simulink model "Revolution_Current_Double_Loop_math"  (Simulink 7.5)
settings: Solver=ode15s  StartTime=0.0  StopTime=6  RelTol=1e-3
libraries: simulink x1, powerlib x1
settings Model: Creator=lm  LastModifiedBy=lm

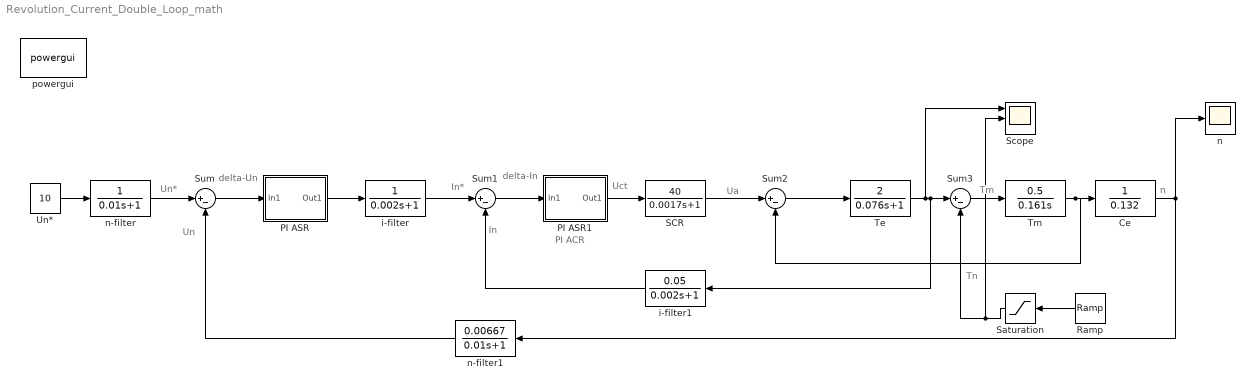
== system Revolution_Current_Double_Loop_math ==
  note: Tm
  note: n
  note: Tn
  note: Un*
  note: Un
  note: delta-Un
  note: In*
  note: In
  note: delta-In
  note: Uct
  note: Ua
  note: PI ACR
  Ce : TransferFcn  Denominator=[0 0.132]
  PI ASR : Subsystem
  PI ASR1 : Subsystem
  Ramp : simulink/Sources/Ramp  SystemSampleTime=-1  slope=1000  start=0.8  X0=0
  SCR : TransferFcn  Numerator=40  Denominator=[0.0017 1]
  Saturation : Saturate  UpperLimit=2222  OutDataType=fixdt(1, 16)  OutScaling=2^0
  Scope : Scope  NumInputPorts=3
      settings: YMin=-5~-5~-5  YMax=5~5~5
  Sum{,1..3} (4 alike) : Sum  Inputs=|+-  OutDataType=fixdt(1, 16)  OutScaling=2^0
  Te : TransferFcn  Numerator=[2]  Denominator=[0.076 1]
  Tm : TransferFcn  Numerator=[0.5]  Denominator=[0.161 0]
  Un* : Constant  Value=10  OutDataType=fixdt(1, 16)  OutScaling=2^0
  i-filter : TransferFcn  Denominator=[0.002 1]
  i-filter1 : TransferFcn  Numerator=0.05  Denominator=[0.002 1]
  n : Scope
  n-filter : TransferFcn  Denominator=[0.01 1]
  n-filter1 : TransferFcn  Numerator=[0.00667]  Denominator=[0.01 1]
  powergui : powerlib/powergui  Priority=1  SystemSampleTime=-1  SimulationMode=Discrete  SampleTime=50e-6  frequency=60  SPID=off  DisableSnubberDevices=off  DisableRonSwitches=off  DisableVfSwitches=off  SwTol=0  Interpol=off  frequencyindice=0  echomessages=off  HookPort=off  DisplayEquations=off  FunctionMessages=off  EnableUseOfTLC=off  x0status=blocks  RestoreLinks=warning  ResistiveCurrentMeasurement=off  Ylog=off  Xlog=on  ShowGrid=off  save=off  variable=ZData  ZoomFFT=off  StartTime=0.0  cycles=1  DisplayStyle=1  FreqAxis=off  MaxFrequency=1000  frequencyindicesteady=1  display=off  methode=off
  wires:
  Un*/1 -> n-filter/1
  n-filter/1 -> Sum/1
  Sum/1 -> PI ASR/1(In1)
  PI ASR/1(Out1) -> i-filter/1
  i-filter/1 -> Sum1/1
  Sum1/1 -> PI ASR1/1(In1)
  PI ASR1/1(Out1) -> SCR/1
  SCR/1 -> Sum2/1
  Te/1 -> Scope/1, Sum3/1, i-filter1/1
  Sum3/1 -> Tm/1
  Tm/1 -> Ce/1, Sum2/2
  Ce/1 -> n/1, n-filter1/1
  i-filter1/1 -> Sum1/2
  Saturation/1 -> Sum3/2, Scope/2
  Ramp/1 -> Saturation/1
  n-filter1/1 -> Sum/2
  Sum2/1 -> Te/1

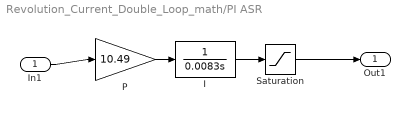
== system Revolution_Current_Double_Loop_math/PI ASR ==
  In1 : Inport
  I : TransferFcn  Denominator=[0.0083 0]  AbsoluteTolerance=12
  P : Gain  Gain=10.49  ParameterDataType=fixdt(1, 16)  ParameterScaling=2^0  OutDataType=fixdt(1, 16)  OutScaling=2^0
  Saturation : Saturate  UpperLimit=10  LowerLimit=-10  OutDataType=fixdt(1, 16)  OutScaling=2^0
  Out1 : Outport
  wires:
  In1/1 -> P/1
  I/1 -> Saturation/1
  Saturation/1 -> Out1/1
  P/1 -> I/1

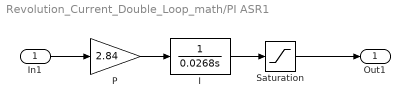
== system Revolution_Current_Double_Loop_math/PI ASR1 ==
  In1 : Inport
  I : TransferFcn  Denominator=[0.0268 0]  AbsoluteTolerance=12
  P : Gain  Gain=2.84  ParameterDataType=fixdt(1, 16)  ParameterScaling=2^0  OutDataType=fixdt(1, 16)  OutScaling=2^0
  Saturation : Saturate  UpperLimit=10  LowerLimit=-10  OutDataType=fixdt(1, 16)  OutScaling=2^0
  Out1 : Outport
  wires:
  P/1 -> I/1
  Saturation/1 -> Out1/1
  I/1 -> Saturation/1
  In1/1 -> P/1
